simulink model "Template_model_32"  (R2024b)
settings: Solver=FixedStepDiscrete  StartTime=0.0  StopTime=10.0  RelTol=1e-3
settings Model: DataTypeOverride=Off  Creator=Mateusz  LastModifiedBy=Mateusz
settings OptimizationCC: BlockReduction=off  ConditionallyExecuteInputs=off  DefaultParameterBehavior=Inlined  InheritOutputTypeSmallerThanSingle=on
settings DebuggingCC: ArtificialAlgebraicLoopMsg=error  SingleTaskRateTransMsg=error
settings HardwareCC: ProdBitPerPointer=32  ProdBitPerSizeT=32  ProdBitPerPtrDiffT=32  ProdLargestAtomicFloat=None  ProdIntDivRoundTo=Undefined  ProdEndianess=Unspecified  ProdWordSize=32  ProdHWDeviceType=ASIC/FPGA->ASIC/FPGA  TargetBitPerPointer=64  TargetBitPerSizeT=64  TargetBitPerPtrDiffT=64  TargetLongLongMode=on  TargetIntDivRoundTo=Zero  TargetEndianess=LittleEndian  TargetWordSize=64  TargetHWDeviceType=Custom Processor->MATLAB Host Computer  ProdEqTarget=off

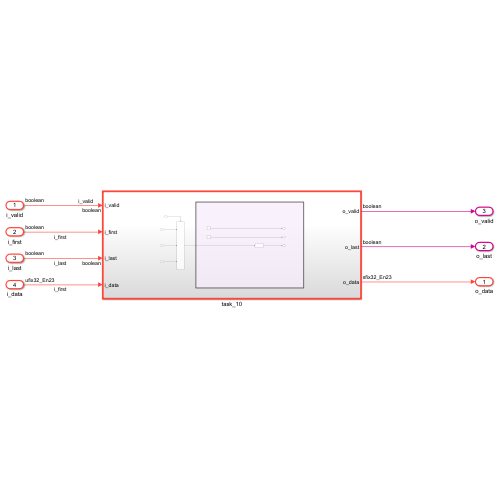
[thumbnail: Simulink's stored preview of the top-level diagram]
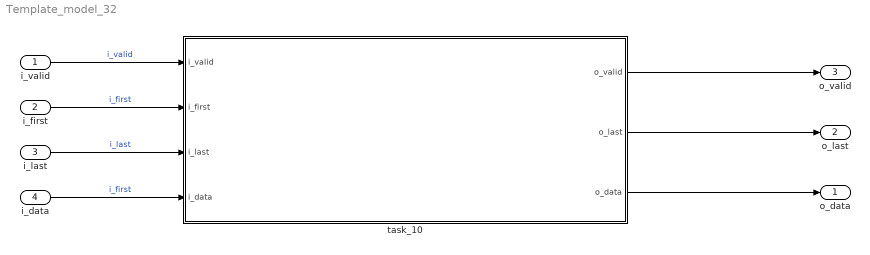
== system Template_model_32 ==
  i_valid : Inport
  i_first : Inport  Port=2
  i_last : Inport  Port=3
  i_data : Inport  Port=4  OutDataTypeStr=fixdt(0,32,23)
  task_10 : Subsystem  TreatAsAtomicUnit=on
  o_data : Outport
  o_last : Outport  Port=2
  o_valid : Outport  Port=3
  wires:
  i_valid/1 -> task_10/1(i_valid)  "i_valid"
  i_first/1 -> task_10/2(i_first)  "i_first"
  i_last/1 -> task_10/3(i_last)  "i_last"
  i_data/1 -> task_10/4(i_data)  "i_first"
  task_10/3(o_data) -> o_data/1
  task_10/2(o_last) -> o_last/1
  task_10/1(o_valid) -> o_valid/1

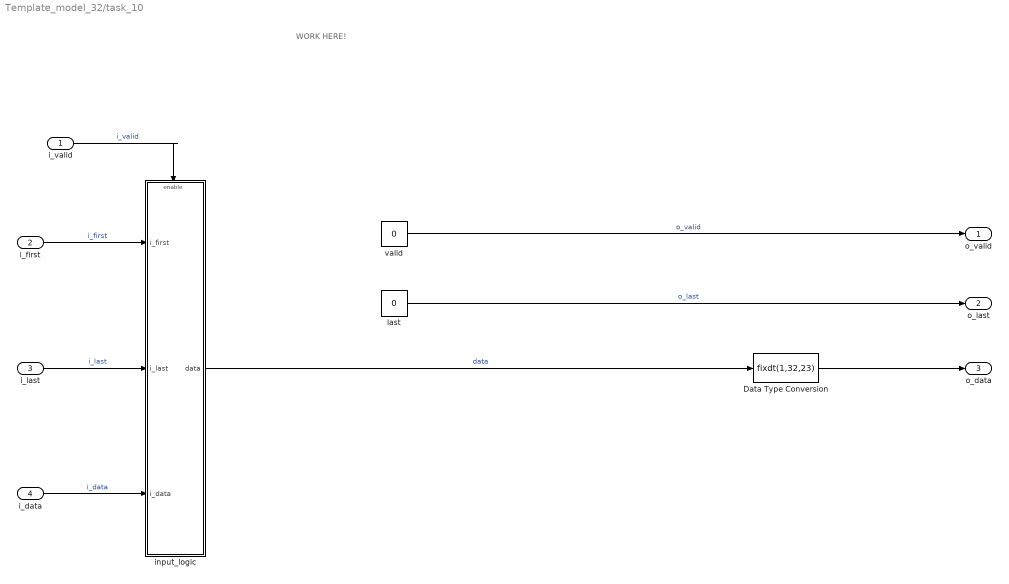
== system Template_model_32/task_10 ==
  note: WORK HERE!
  i_valid : Inport  OutDataTypeStr=boolean
  i_first : Inport  Port=2
  i_last : Inport  Port=3  OutDataTypeStr=boolean
  i_data : Inport  Port=4
  Data Type Conversion : DataTypeConversion  OutDataTypeStr=fixdt(1,32,23)  SaturateOnIntegerOverflow=off  RndMeth=Floor
  input_logic : Subsystem
  last : Constant  Value=0  OutDataTypeStr=boolean
  valid : Constant  Value=0  OutDataTypeStr=boolean
  o_valid : Outport
  o_last : Outport  Port=2
  o_data : Outport  Port=3
  wires:
  i_first/1 -> input_logic/1(i_first)  "i_first"
  i_last/1 -> input_logic/2(i_last)  "i_last"
  i_data/1 -> input_logic/3(i_data)  "i_data"
  i_valid/1 -> input_logic/Enable  "i_valid"
  input_logic/1(data) -> Data Type Conversion/1  "data"
  last/1 -> o_last/1  "o_last"
  valid/1 -> o_valid/1  "o_valid"
  Data Type Conversion/1 -> o_data/1

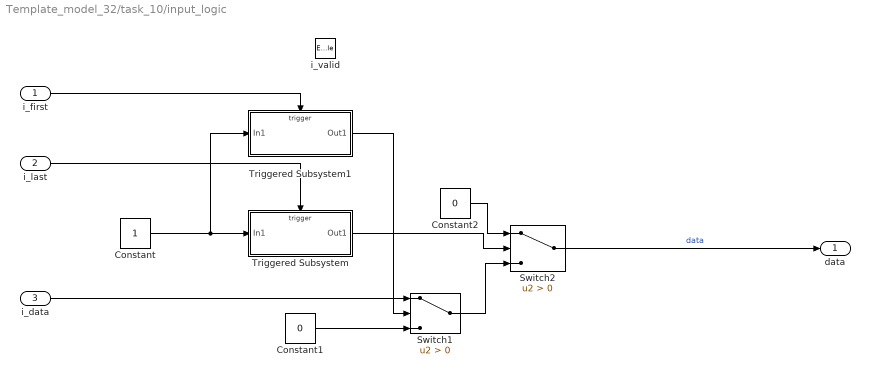
== system Template_model_32/task_10/input_logic ==
  i_first : Inport  OutDataTypeStr=boolean
  i_last : Inport  Port=2
  i_data : Inport  Port=3
  i_valid : EnablePort
  Constant : Constant  OutDataTypeStr=boolean
  Constant1 : Constant  Value=0  OutDataTypeStr=fixdt(0,32,23)
  Constant2 : Constant  Value=0  OutDataTypeStr=fixdt(0,32,23)
  Switch1 : Switch  Criteria=u2 > Threshold  SaturateOnIntegerOverflow=off  InputSameDT=off
  Switch2 : Switch  Criteria=u2 > Threshold  SaturateOnIntegerOverflow=off  InputSameDT=off
  Triggered Subsystem : Subsystem  TreatAsAtomicUnit=on
  Triggered Subsystem1 : Subsystem  TreatAsAtomicUnit=on
  data : Outport
  wires:
  Constant/1 -> Triggered Subsystem/1(In1), Triggered Subsystem1/1(In1)
  Triggered Subsystem1/1(Out1) -> Switch1/2
  i_last/1 -> Triggered Subsystem/Trigger
  Constant1/1 -> Switch1/3
  Triggered Subsystem/1(Out1) -> Switch2/2
  Switch2/1 -> data/1  "data"
  Switch1/1 -> Switch2/3
  i_first/1 -> Triggered Subsystem1/Trigger
  i_data/1 -> Switch1/1
  Constant2/1 -> Switch2/1

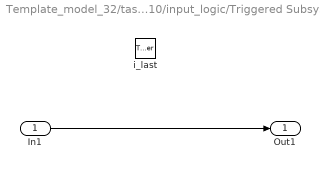
== system Template_model_32/task_10/input_logic/Triggered Subsystem ==
  In1 : Inport
  i_last : TriggerPort  TriggerType=falling  VariantControl=(inherit)
  Out1 : Outport  InitialOutput=0
  wires:
  In1/1 -> Out1/1

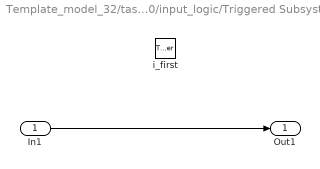
== system Template_model_32/task_10/input_logic/Triggered Subsystem1 ==
  In1 : Inport
  i_first : TriggerPort  VariantControl=(inherit)
  Out1 : Outport  InitialOutput=0
  wires:
  In1/1 -> Out1/1
